simulink model "Coupled_Model_crosslinked_intext"  (R2016a)
settings: Solver=FixedStepDiscrete  StartTime=0  StopTime=1000  FixedStep=1  RelTol=1e-3
undefined symbols (not defined in the file or in its folder): DiscIntNeverNeededParam
libraries: simulink_extras x32
(part 1 of 3)
settings Model: Creator=bloomlab  LastModifiedBy=lawrimor
settings SolverCC: MaxOrder=2  AlgebraicLoopSolver=LineSearch
settings DataIOCC: LimitDataPoints=on  SaveFormat=Array  SignalLoggingSaveFormat=ModelDataLogs
settings OptimizationCC: ExpressionDepthLimit=2147483647  InitFltsAndDblsToZero=on
settings DebuggingCC: UnderspecifiedInitializationDetection=Classic  MergeDetectMultiDrivingBlocksExec=none  SolverPrmCheckMsg=warning  FcnCallInpInsideContextMsg=UseLocalSettings  UnconnectedOutputMsg=none  StateNameClashWarn=warning  StrictBusMsg=Warning
settings HardwareCC: ProdBitPerPointer=32  ProdLargestAtomicFloat=None  ProdIntDivRoundTo=Undefined  ProdEndianess=Unspecified  ProdWordSize=32  ProdHWDeviceType=32-bit Generic
settings ModelReferenceCC: ModelReferenceMinAlgLoopOccurrences=on  PropagateSignalLabelsOutOfModel=off
settings GRTTargetCC: CombineOutputUpdateFcns=off  GRTInterface=on
settings ConfigComp: CovModelRefEnable=Off

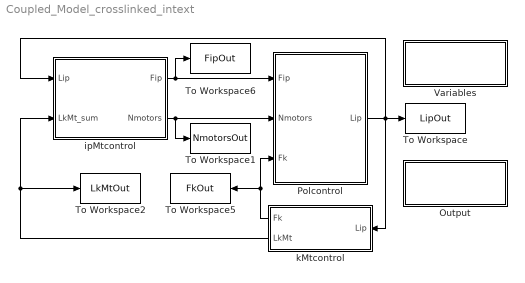
== system Coupled_Model_crosslinked_intext ==
  Output : Subsystem
  Polcontrol : Subsystem
  To Workspace : ToWorkspace  VariableName=LipOut  SampleTime=-1
  To Workspace1 : ToWorkspace  VariableName=NmotorsOut  SampleTime=-1
  To Workspace2 : ToWorkspace  VariableName=LkMtOut  SampleTime=-1
  To Workspace5 : ToWorkspace  VariableName=FkOut  SampleTime=-1
  To Workspace6 : ToWorkspace  VariableName=FipOut  SampleTime=-1
  Variables : Subsystem
  ipMtcontrol : Subsystem
  kMtcontrol : Subsystem
  wires:
  ipMtcontrol/2(Nmotors) -> Polcontrol/2(Nmotors), To Workspace1/1
  ipMtcontrol/1(Fip) -> Polcontrol/1(Fip), To Workspace6/1
  kMtcontrol/1(Fk) -> To Workspace5/1, Polcontrol/3(Fk)
  kMtcontrol/2(LkMt) -> ipMtcontrol/2(LkMt_sum), To Workspace2/1
  Polcontrol/1(Lip) -> kMtcontrol/1(Lip), ipMtcontrol/1(Lip), To Workspace/1

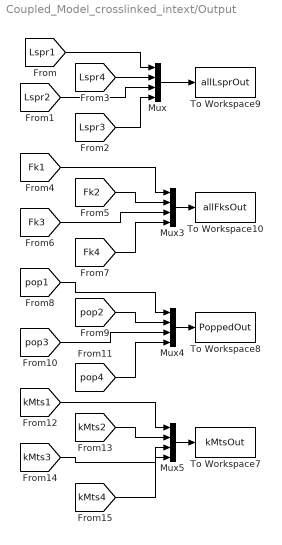
== system Coupled_Model_crosslinked_intext/Output ==
  Mux{,3..5} (4 alike) : Mux
  To Workspace10 : ToWorkspace  VariableName=allFksOut  SampleTime=-1
  To Workspace7 : ToWorkspace  VariableName=kMtsOut  SampleTime=-1
  To Workspace8 : ToWorkspace  VariableName=PoppedOut  SampleTime=-1
  To Workspace9 : ToWorkspace  VariableName=allLsprOut  SampleTime=-1
  wires:
  Mux/1 -> To Workspace9/1
  [Lspr1] -> Mux/1
  [Lspr4] -> Mux/2
  [Lspr2] -> Mux/3
  [Lspr3] -> Mux/4
  Mux3/1 -> To Workspace10/1
  [Fk1] -> Mux3/1
  [Fk2] -> Mux3/2
  [Fk3] -> Mux3/3
  [Fk4] -> Mux3/4
  Mux4/1 -> To Workspace8/1
  [pop1] -> Mux4/1
  [pop2] -> Mux4/2
  [pop3] -> Mux4/3
  [pop4] -> Mux4/4
  Mux5/1 -> To Workspace7/1
  [kMts1] -> Mux5/1
  [kMts2] -> Mux5/2
  [kMts3] -> Mux5/3
  [kMts4] -> Mux5/4

== system Coupled_Model_crosslinked_intext/Polcontrol ==
  Fip : Inport
  Nmotors : Inport  Port=2
  Fk : Inport  Port=3
  Discrete-Time Integrator : DiscreteIntegrator  InitialConditionSource=external  InitialCondition=1.5e-6  ICPrevOutput=DiscIntNeverNeededParam  ICPrevScaledInput=DiscIntNeverNeededParam
  Embedded MATLAB Function : MATLAB Function  TreatAsAtomicUnit=on
  Embedded MATLAB Function1 : MATLAB Function  TreatAsAtomicUnit=on
  Embedded MATLAB Function2 : MATLAB Function  TreatAsAtomicUnit=on
  Embedded MATLAB Function3 : MATLAB Function  TreatAsAtomicUnit=on
  Product : Product  RndMeth=Zero
  Sum : Sum
  Sum1 : Sum
  To Workspace4 : ToWorkspace  VariableName=vipOut  SampleTime=-1
  Lip : Outport
  wires:
  Embedded MATLAB Function/1(Vip) -> Product/1
  Fip/1 -> Sum/1
  Sum/1 -> Embedded MATLAB Function1/1(Fnet), Sum1/1
  Embedded MATLAB Function1/1(y) -> Embedded MATLAB Function/1(Fnet)
  Sum1/1 -> Embedded MATLAB Function3/1(Fnet)
  Embedded MATLAB Function3/1(y) -> Embedded MATLAB Function2/1(Fnet)
  Product/1 -> Sum1/2
  Embedded MATLAB Function2/1(Vip) -> Discrete-Time Integrator/1, To Workspace4/1
  Discrete-Time Integrator/1 -> Lip/1
  Nmotors/1 -> Embedded MATLAB Function1/2(Nmotors), Embedded MATLAB Function3/2(Nmotors)
  Fk/1 -> Sum/2
  [Cd] -> Product/2
  [Lip] -> Discrete-Time Integrator/2

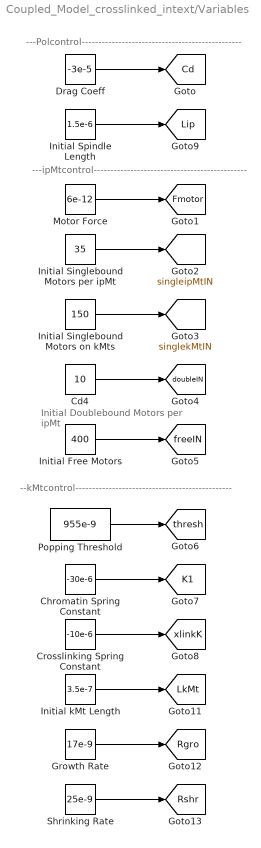
== system Coupled_Model_crosslinked_intext/Variables ==
  note: ---Polcontrol------------------------------------------------
  note: ---ipMtcontrol----------------------------------------------
  note: Initial Doublebound
      | Motors per ipMt
  note: --kMtcontrol-----------------------------------------------
  Cd4 : Constant  Value=10
  Chromatin Spring Constant : Constant  Value=-30e-6
  Crosslinking Spring Constant : Constant  Value=-10e-6
  Drag Coeff : Constant  Value=-3e-5
  Growth Rate : Constant  Value=17e-9
  Initial Free Motors : Constant  Value=400
  Initial Singlebound Motors on kMts : Constant  Value=150
  Initial Singlebound Motors per ipMt : Constant  Value=35
  Initial Spindle Length : Constant  Value=1.5e-6
  Initial kMt Length : Constant  Value=3.5e-7
  Motor Force : Constant  Value=6e-12
  Popping Threshold : Constant  Value=955e-9
  Shrinking Rate : Constant  Value=25e-9
  tag scope: Cd=global, Fmotor=global, K1=global, Lip=global, LkMt=global, Rgro=global, Rshr=global, doubleIN=global, freeIN=global, singleipMtIN=global, singlekMtIN=global, thresh=global, xlinkK=global
  wires:
  Drag Coeff/1 -> [Cd]
  Motor Force/1 -> [Fmotor]
  Initial Singlebound Motors per ipMt/1 -> [singleipMtIN]
  Initial Singlebound Motors on kMts/1 -> [singlekMtIN]
  Cd4/1 -> [doubleIN]
  Initial Free Motors/1 -> [freeIN]
  Popping Threshold/1 -> [thresh]
  Chromatin Spring Constant/1 -> [K1]
  Crosslinking Spring Constant/1 -> [xlinkK]
  Initial Spindle Length/1 -> [Lip]
  Initial kMt Length/1 -> [LkMt]
  Growth Rate/1 -> [Rgro]
  Shrinking Rate/1 -> [Rshr]

== system Coupled_Model_crosslinked_intext/ipMtcontrol ==
  note: Fk
  Lip : Inport
  LkMt_sum : Inport  Port=2
  Constant : Constant  Value=0.8e-6
  Embedded MATLAB Function1 : MATLAB Function
  Product : Product  RndMeth=Zero
  To Workspace3 : ToWorkspace  VariableName=LlapOut  SampleTime=-1
  Fip : Outport
  Nmotors : Outport  Port=2
  wires:
  Lip/1 -> Embedded MATLAB Function1/5(Lip)
  LkMt_sum/1 -> Embedded MATLAB Function1/7(LkMt)
  Product/1 -> Fip/1
  Embedded MATLAB Function1/1(Nmotors) -> Nmotors/1, Product/1
  [Fmotor] -> Product/2
  [singleipMtIN] -> Embedded MATLAB Function1/1(singleipMtIN)
  [singlekMtIN] -> Embedded MATLAB Function1/2(singlekMtIN)
  [doubleIN] -> Embedded MATLAB Function1/3(doubleIN)
  [freeIN] -> Embedded MATLAB Function1/4(freeIN)
  Constant/1 -> Embedded MATLAB Function1/6(Llap), To Workspace3/1

== system Coupled_Model_crosslinked_intext/kMtcontrol ==
  Lip : Inport
  Sum : Sum  Inputs=++++
  Sum1 : Sum  Inputs=++++
  kMtcontrol : Subsystem
  kMtcontrol1 : Subsystem
  kMtcontrol2 : Subsystem
  kMtcontrol3 : Subsystem
  Fk : Outport
  LkMt : Outport  Port=2
  wires:
  kMtcontrol/1(LkMt_sum) -> Sum/1
  kMtcontrol1/1(LkMt_sum) -> Sum/2
  kMtcontrol2/1(LkMt_sum) -> Sum/3
  kMtcontrol3/1(LkMt_sum) -> Sum/4
  kMtcontrol/2(Fk) -> Sum1/1
  kMtcontrol1/2(Fk) -> Sum1/2
  kMtcontrol2/2(Fk) -> Sum1/3
  kMtcontrol3/2(Fk) -> Sum1/4
  kMtcontrol/3(Lspring4) -> kMtcontrol1/2(Lspring4)
  kMtcontrol1/3(Lspring8) -> kMtcontrol2/2(Lspring8)
  kMtcontrol2/3(Lspring12) -> kMtcontrol3/2(Lspring12)
  kMtcontrol/4(Lspring1) -> kMtcontrol3/3(Lspring1)
  kMtcontrol3/4(Lspring13) -> kMtcontrol2/3(Lspring13)
  kMtcontrol2/4(Lspring9) -> kMtcontrol1/3(Lspring9)
  kMtcontrol1/4(Lspring5) -> kMtcontrol/3(Lspring5)
  kMtcontrol3/3(Lspring16) -> kMtcontrol/2(Lspring16)
  Lip/1 -> kMtcontrol2/1("Lip "), kMtcontrol3/1("Lip "), kMtcontrol/1("Lip "), kMtcontrol1/1("Lip ")
  Sum/1 -> LkMt/1
  Sum1/1 -> Fk/1

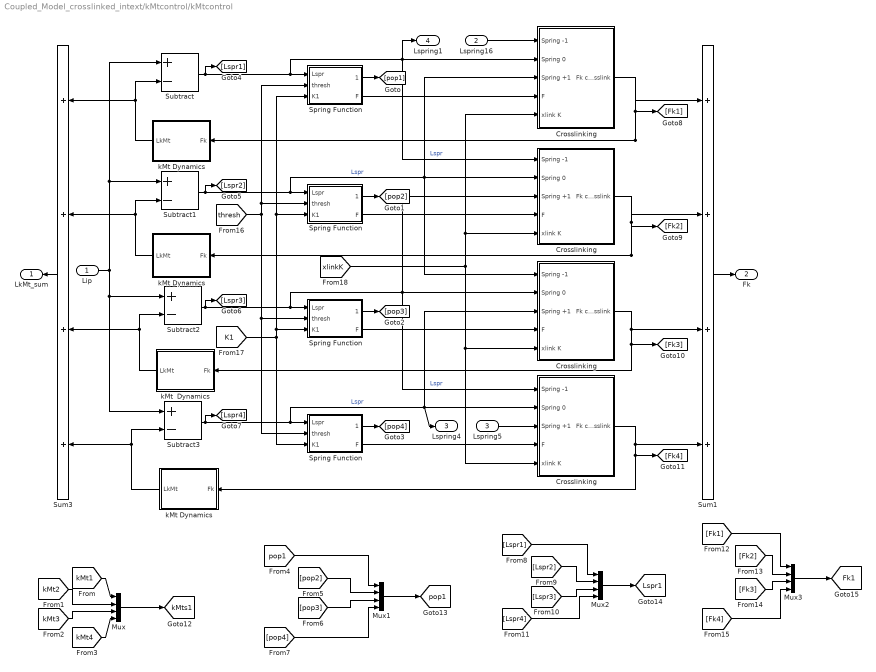
== system Coupled_Model_crosslinked_intext/kMtcontrol/kMtcontrol ==
  "Lip " : Inport
  Lspring16 : Inport  Port=2
  Lspring5 : Inport  Port=3
  " Crosslinking  " : Subsystem
  " Spring Function" : MATLAB Function  TreatAsAtomicUnit=on
  " Spring Function " : MATLAB Function  TreatAsAtomicUnit=on
  "Crosslinking " : Subsystem
  "Crosslinking  " : Subsystem
  "Crosslinking   " : Subsystem
  Mux{,1..3} (4 alike) : Mux
  Spring Function : MATLAB Function  TreatAsAtomicUnit=on
  "Spring Function " : MATLAB Function  TreatAsAtomicUnit=on
  Subtract{,1..3} (4 alike) : Sum  Inputs=+-
  Sum1 : Sum  Inputs=++++
  Sum3 : Sum  Inputs=++++
  kMt  Dynamics : Subsystem
  kMt Dynamics : Subsystem
  "kMt Dynamics " : Subsystem
  "kMt Dynamics  " : Subsystem
  LkMt_sum : Outport
  Fk : Outport  Port=2
  Lspring4 : Outport  Port=3
  Lspring1 : Outport  Port=4
  tag scope: Fk1=global, Lspr1=global, kMts1=global, pop1=global
  wires:
  "kMt Dynamics  "/1(LkMt) -> Subtract3/2, Sum3/4
  kMt  Dynamics/1(LkMt) -> Subtract2/2, Sum3/3
  "kMt Dynamics "/1(LkMt) -> Sum3/2, Subtract1/2
  kMt Dynamics/1(LkMt) -> Subtract/2, Sum3/1
  "Lip "/1 -> Subtract/1, Subtract1/1, Subtract2/1, Subtract3/1
  Sum1/1 -> Fk/1
  Subtract/1 -> [Lspr1], Spring Function/1(Lspr), "Crosslinking "/1(Spring -1), Lspring1/1, "Crosslinking  "/2(Spring 0)  "Lspr"
  Subtract1/1 -> [Lspr2], "Crosslinking  "/3(Spring +1), "Crosslinking "/2(Spring 0), " Crosslinking  "/1(Spring -1), "Spring Function "/1(Lspr)  "Lspr"
  Subtract2/1 -> [Lspr3], " Spring Function"/1(Lspr), " Crosslinking  "/2(Spring 0), "Crosslinking "/3(Spring +1), "Crosslinking   "/1(Spring -1)  "Lspr"
  Subtract3/1 -> [Lspr4], "Crosslinking   "/2(Spring 0), " Crosslinking  "/3(Spring +1), Lspring4/1, " Spring Function "/1(Lspr)  "Lspr"
  Spring Function/1(popped) -> [pop1]
  "Spring Function "/1(popped) -> [pop2]
  " Spring Function"/1(popped) -> [pop3]
  " Spring Function "/1(popped) -> [pop4]
  Mux/1 -> [kMts1]
  [kMt1] -> Mux/1
  [kMt2] -> Mux/2
  [kMt3] -> Mux/3
  [kMt4] -> Mux/4
  [pop1] -> Mux1/1
  [pop2] -> Mux1/2
  [pop3] -> Mux1/3
  [pop4] -> Mux1/4
  Mux1/1 -> [pop1]
  Mux2/1 -> [Lspr1]
  [Lspr1] -> Mux2/1
  [Lspr2] -> Mux2/2
  [Lspr3] -> Mux2/3
  [Lspr4] -> Mux2/4
  Mux3/1 -> [Fk1]
  [Fk1] -> Mux3/1
  [Fk2] -> Mux3/2
  [Fk3] -> Mux3/3
  [Fk4] -> Mux3/4
  Spring Function/2(F) -> "Crosslinking  "/4(F)
  "Crosslinking  "/1(Fk crosslink) -> kMt Dynamics/1(Fk), Sum1/1, [Fk1]
  "Spring Function "/2(F) -> "Crosslinking "/4(F)
  "Crosslinking "/1(Fk crosslink) -> Sum1/2, "kMt Dynamics "/1(Fk), [Fk2]
  " Spring Function"/2(F) -> " Crosslinking  "/4(F)
  " Crosslinking  "/1(Fk crosslink) -> [Fk3], kMt  Dynamics/1(Fk), Sum1/3
  " Spring Function "/2(F) -> "Crosslinking   "/4(F)
  "Crosslinking   "/1(Fk crosslink) -> Sum1/4, [Fk4], "kMt Dynamics  "/1(Fk)
  Lspring16/1 -> "Crosslinking  "/1(Spring -1)
  Lspring5/1 -> "Crosslinking   "/3(Spring +1)
  Sum3/1 -> LkMt_sum/1
  [thresh] -> "Spring Function "/2(thresh), Spring Function/2(thresh), " Spring Function"/2(thresh), " Spring Function "/2(thresh)
  [xlinkK] -> "Crosslinking "/5(xlink K), "Crosslinking  "/5(xlink K), " Crosslinking  "/5(xlink K), "Crosslinking   "/5(xlink K)
  [K1] -> " Spring Function "/3(K1), " Spring Function"/3(K1), "Spring Function "/3(K1), Spring Function/3(K1)

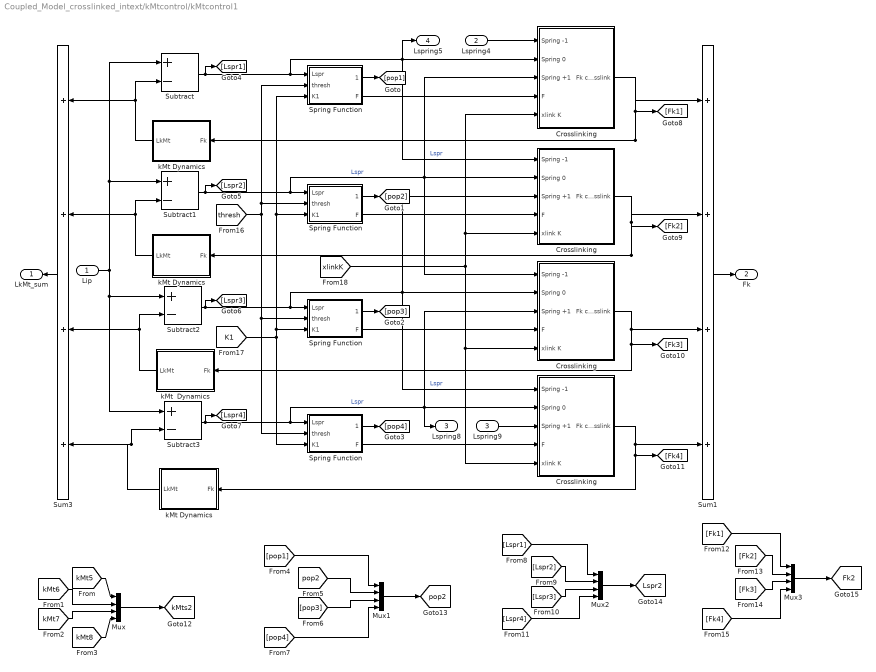
== system Coupled_Model_crosslinked_intext/kMtcontrol/kMtcontrol1 ==
  "Lip " : Inport
  Lspring4 : Inport  Port=2
  Lspring9 : Inport  Port=3
  " Crosslinking  " : Subsystem
  " Spring Function" : MATLAB Function  TreatAsAtomicUnit=on
  " Spring Function " : MATLAB Function  TreatAsAtomicUnit=on
  "Crosslinking " : Subsystem
  "Crosslinking  " : Subsystem
  "Crosslinking   " : Subsystem
  Mux{,1..3} (4 alike) : Mux
  Spring Function : MATLAB Function  TreatAsAtomicUnit=on
  "Spring Function " : MATLAB Function  TreatAsAtomicUnit=on
  Subtract{,1..3} (4 alike) : Sum  Inputs=+-
  Sum1 : Sum  Inputs=++++
  Sum3 : Sum  Inputs=++++
  kMt  Dynamics : Subsystem
  kMt Dynamics : Subsystem
  "kMt Dynamics " : Subsystem
  "kMt Dynamics  " : Subsystem
  LkMt_sum : Outport
  Fk : Outport  Port=2
  Lspring8 : Outport  Port=3
  Lspring5 : Outport  Port=4
  tag scope: Fk2=global, Lspr2=global, kMts2=global, pop2=global
  wires:
  [K1] -> " Spring Function "/3(K1), " Spring Function"/3(K1), "Spring Function "/3(K1), Spring Function/3(K1)
  [xlinkK] -> "Crosslinking "/5(xlink K), "Crosslinking  "/5(xlink K), " Crosslinking  "/5(xlink K), "Crosslinking   "/5(xlink K)
  [thresh] -> "Spring Function "/2(thresh), Spring Function/2(thresh), " Spring Function"/2(thresh), " Spring Function "/2(thresh)
  Sum3/1 -> LkMt_sum/1
  Lspring9/1 -> "Crosslinking   "/3(Spring +1)
  Lspring4/1 -> "Crosslinking  "/1(Spring -1)
  "Crosslinking   "/1(Fk crosslink) -> Sum1/4, [Fk4], "kMt Dynamics  "/1(Fk)
  " Spring Function "/2(F) -> "Crosslinking   "/4(F)
  " Crosslinking  "/1(Fk crosslink) -> [Fk3], kMt  Dynamics/1(Fk), Sum1/3
  " Spring Function"/2(F) -> " Crosslinking  "/4(F)
  "Crosslinking "/1(Fk crosslink) -> Sum1/2, "kMt Dynamics "/1(Fk), [Fk2]
  "Spring Function "/2(F) -> "Crosslinking "/4(F)
  "Crosslinking  "/1(Fk crosslink) -> Sum1/1, kMt Dynamics/1(Fk), [Fk1]
  Spring Function/2(F) -> "Crosslinking  "/4(F)
  [Fk4] -> Mux3/4
  [Fk3] -> Mux3/3
  [Fk2] -> Mux3/2
  [Fk1] -> Mux3/1
  Mux3/1 -> [Fk2]
  [Lspr4] -> Mux2/4
  [Lspr3] -> Mux2/3
  [Lspr2] -> Mux2/2
  [Lspr1] -> Mux2/1
  Mux2/1 -> [Lspr2]
  Mux1/1 -> [pop2]
  [pop4] -> Mux1/4
  [pop3] -> Mux1/3
  [pop2] -> Mux1/2
  [pop1] -> Mux1/1
  [kMt8] -> Mux/4
  [kMt7] -> Mux/3
  [kMt6] -> Mux/2
  [kMt5] -> Mux/1
  Mux/1 -> [kMts2]
  " Spring Function "/1(popped) -> [pop4]
  " Spring Function"/1(popped) -> [pop3]
  "Spring Function "/1(popped) -> [pop2]
  Spring Function/1(popped) -> [pop1]
  Subtract3/1 -> [Lspr4], "Crosslinking   "/2(Spring 0), " Crosslinking  "/3(Spring +1), Lspring8/1, " Spring Function "/1(Lspr)  "Lspr"
  Subtract2/1 -> [Lspr3], " Spring Function"/1(Lspr), " Crosslinking  "/2(Spring 0), "Crosslinking "/3(Spring +1), "Crosslinking   "/1(Spring -1)  "Lspr"
  Subtract1/1 -> [Lspr2], "Crosslinking  "/3(Spring +1), "Crosslinking "/2(Spring 0), " Crosslinking  "/1(Spring -1), "Spring Function "/1(Lspr)  "Lspr"
  Subtract/1 -> [Lspr1], Spring Function/1(Lspr), "Crosslinking "/1(Spring -1), Lspring5/1, "Crosslinking  "/2(Spring 0)  "Lspr"
  Sum1/1 -> Fk/1
  "Lip "/1 -> Subtract/1, Subtract1/1, Subtract2/1, Subtract3/1
  kMt Dynamics/1(LkMt) -> Subtract/2, Sum3/1
  "kMt Dynamics "/1(LkMt) -> Sum3/2, Subtract1/2
  kMt  Dynamics/1(LkMt) -> Subtract2/2, Sum3/3
  "kMt Dynamics  "/1(LkMt) -> Subtract3/2, Sum3/4

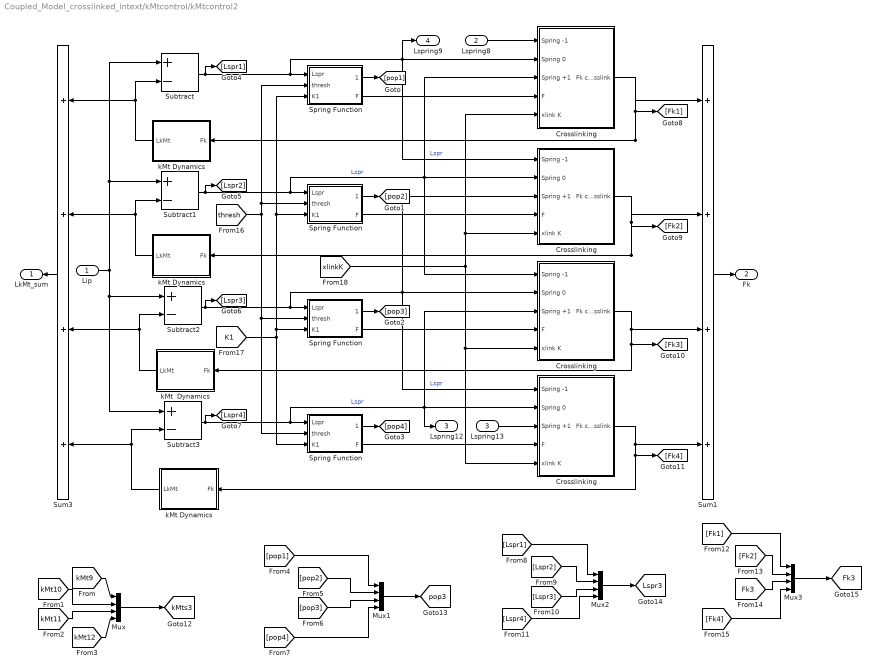
== system Coupled_Model_crosslinked_intext/kMtcontrol/kMtcontrol2 ==
  "Lip " : Inport
  Lspring8 : Inport  Port=2
  Lspring13 : Inport  Port=3
  " Crosslinking  " : Subsystem
  " Spring Function" : MATLAB Function  TreatAsAtomicUnit=on
  " Spring Function " : MATLAB Function  TreatAsAtomicUnit=on
  "Crosslinking " : Subsystem
  "Crosslinking  " : Subsystem
  "Crosslinking   " : Subsystem
  Mux{,1..3} (4 alike) : Mux
  Spring Function : MATLAB Function  TreatAsAtomicUnit=on
  "Spring Function " : MATLAB Function  TreatAsAtomicUnit=on
  Subtract{,1..3} (4 alike) : Sum  Inputs=+-
  Sum1 : Sum  Inputs=++++
  Sum3 : Sum  Inputs=++++
  kMt  Dynamics : Subsystem
  kMt Dynamics : Subsystem
  "kMt Dynamics " : Subsystem
  "kMt Dynamics  " : Subsystem
  LkMt_sum : Outport
  Fk : Outport  Port=2
  Lspring12 : Outport  Port=3
  Lspring9 : Outport  Port=4
  tag scope: Fk3=global, Lspr3=global, kMts3=global, pop3=global
  wires:
  "kMt Dynamics  "/1(LkMt) -> Subtract3/2, Sum3/4
  kMt  Dynamics/1(LkMt) -> Subtract2/2, Sum3/3
  "kMt Dynamics "/1(LkMt) -> Sum3/2, Subtract1/2
  kMt Dynamics/1(LkMt) -> Subtract/2, Sum3/1
  "Lip "/1 -> Subtract/1, Subtract1/1, Subtract2/1, Subtract3/1
  Sum1/1 -> Fk/1
  Subtract/1 -> [Lspr1], Spring Function/1(Lspr), "Crosslinking "/1(Spring -1), Lspring9/1, "Crosslinking  "/2(Spring 0)  "Lspr"
  Subtract1/1 -> [Lspr2], "Crosslinking  "/3(Spring +1), "Crosslinking "/2(Spring 0), " Crosslinking  "/1(Spring -1), "Spring Function "/1(Lspr)  "Lspr"
  Subtract2/1 -> [Lspr3], " Spring Function"/1(Lspr), " Crosslinking  "/2(Spring 0), "Crosslinking "/3(Spring +1), "Crosslinking   "/1(Spring -1)  "Lspr"
  Subtract3/1 -> [Lspr4], "Crosslinking   "/2(Spring 0), " Crosslinking  "/3(Spring +1), Lspring12/1, " Spring Function "/1(Lspr)  "Lspr"
  Spring Function/1(popped) -> [pop1]
  "Spring Function "/1(popped) -> [pop2]
  " Spring Function"/1(popped) -> [pop3]
  " Spring Function "/1(popped) -> [pop4]
  Mux/1 -> [kMts3]
  [kMt9] -> Mux/1
  [kMt10] -> Mux/2
  [kMt11] -> Mux/3
  [kMt12] -> Mux/4
  [pop1] -> Mux1/1
  [pop2] -> Mux1/2
  [pop3] -> Mux1/3
  [pop4] -> Mux1/4
  Mux1/1 -> [pop3]
  Mux2/1 -> [Lspr3]
  [Lspr1] -> Mux2/1
  [Lspr2] -> Mux2/2
  [Lspr3] -> Mux2/3
  [Lspr4] -> Mux2/4
  Mux3/1 -> [Fk3]
  [Fk1] -> Mux3/1
  [Fk2] -> Mux3/2
  [Fk3] -> Mux3/3
  [Fk4] -> Mux3/4
  Spring Function/2(F) -> "Crosslinking  "/4(F)
  "Crosslinking  "/1(Fk crosslink) -> Sum1/1, kMt Dynamics/1(Fk), [Fk1]
  "Spring Function "/2(F) -> "Crosslinking "/4(F)
  "Crosslinking "/1(Fk crosslink) -> Sum1/2, "kMt Dynamics "/1(Fk), [Fk2]
  " Spring Function"/2(F) -> " Crosslinking  "/4(F)
  " Crosslinking  "/1(Fk crosslink) -> [Fk3], kMt  Dynamics/1(Fk), Sum1/3
  " Spring Function "/2(F) -> "Crosslinking   "/4(F)
  "Crosslinking   "/1(Fk crosslink) -> Sum1/4, [Fk4], "kMt Dynamics  "/1(Fk)
  Lspring8/1 -> "Crosslinking  "/1(Spring -1)
  Lspring13/1 -> "Crosslinking   "/3(Spring +1)
  Sum3/1 -> LkMt_sum/1
  [thresh] -> "Spring Function "/2(thresh), Spring Function/2(thresh), " Spring Function"/2(thresh), " Spring Function "/2(thresh)
  [xlinkK] -> "Crosslinking "/5(xlink K), "Crosslinking  "/5(xlink K), " Crosslinking  "/5(xlink K), "Crosslinking   "/5(xlink K)
  [K1] -> " Spring Function "/3(K1), " Spring Function"/3(K1), "Spring Function "/3(K1), Spring Function/3(K1)

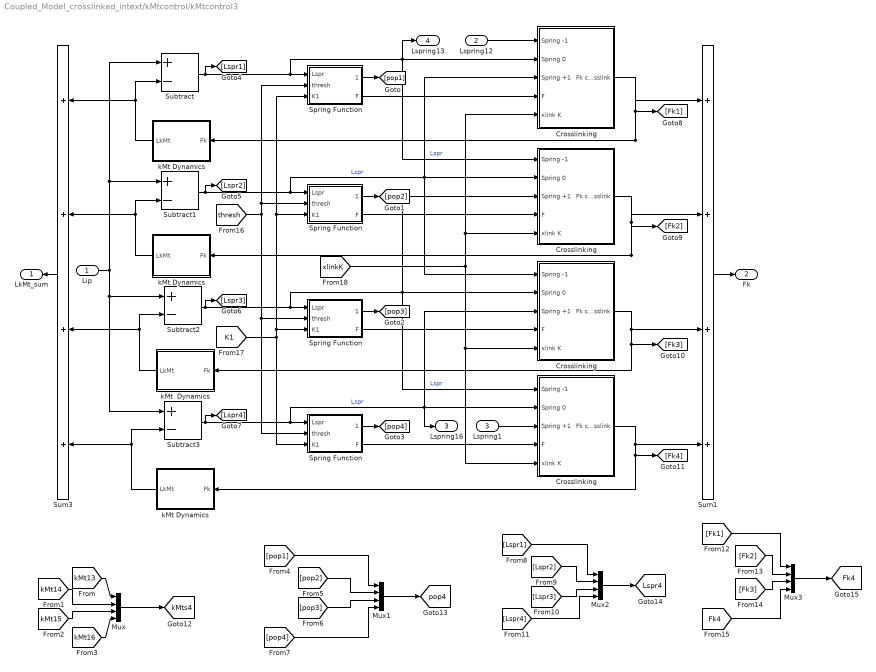
== system Coupled_Model_crosslinked_intext/kMtcontrol/kMtcontrol3 ==
  "Lip " : Inport
  Lspring12 : Inport  Port=2
  Lspring1 : Inport  Port=3
  " Crosslinking  " : Subsystem
  " Spring Function" : MATLAB Function  TreatAsAtomicUnit=on
  " Spring Function " : MATLAB Function  TreatAsAtomicUnit=on
  "Crosslinking " : Subsystem
  "Crosslinking  " : Subsystem
  "Crosslinking   " : Subsystem
  Mux{,1..3} (4 alike) : Mux
  Spring Function : MATLAB Function  TreatAsAtomicUnit=on
  "Spring Function " : MATLAB Function  TreatAsAtomicUnit=on
  Subtract{,1..3} (4 alike) : Sum  Inputs=+-
  Sum1 : Sum  Inputs=++++
  Sum3 : Sum  Inputs=++++
  kMt  Dynamics : Subsystem
  kMt Dynamics : Subsystem
  "kMt Dynamics " : Subsystem
  "kMt Dynamics  " : Subsystem
  LkMt_sum : Outport
  Fk : Outport  Port=2
  Lspring16 : Outport  Port=3
  Lspring13 : Outport  Port=4
  tag scope: Fk4=global, Lspr4=global, kMts4=global, pop4=global
  wires:
  "kMt Dynamics  "/1(LkMt) -> Subtract3/2, Sum3/4
  kMt  Dynamics/1(LkMt) -> Subtract2/2, Sum3/3
  "kMt Dynamics "/1(LkMt) -> Sum3/2, Subtract1/2
  kMt Dynamics/1(LkMt) -> Subtract/2, Sum3/1
  "Lip "/1 -> Subtract/1, Subtract1/1, Subtract2/1, Subtract3/1
  Sum1/1 -> Fk/1
  Subtract/1 -> [Lspr1], Spring Function/1(Lspr), "Crosslinking "/1(Spring -1), Lspring13/1, "Crosslinking  "/2(Spring 0)  "Lspr"
  Subtract1/1 -> [Lspr2], "Crosslinking  "/3(Spring +1), "Crosslinking "/2(Spring 0), " Crosslinking  "/1(Spring -1), "Spring Function "/1(Lspr)  "Lspr"
  Subtract2/1 -> [Lspr3], " Spring Function"/1(Lspr), " Crosslinking  "/2(Spring 0), "Crosslinking "/3(Spring +1), "Crosslinking   "/1(Spring -1)  "Lspr"
  Subtract3/1 -> [Lspr4], "Crosslinking   "/2(Spring 0), " Crosslinking  "/3(Spring +1), Lspring16/1, " Spring Function "/1(Lspr)  "Lspr"
  Spring Function/1(popped) -> [pop1]
  "Spring Function "/1(popped) -> [pop2]
  " Spring Function"/1(popped) -> [pop3]
  " Spring Function "/1(popped) -> [pop4]
  Mux/1 -> [kMts4]
  [kMt13] -> Mux/1
  [kMt14] -> Mux/2
  [kMt15] -> Mux/3
  [kMt16] -> Mux/4
  [pop1] -> Mux1/1
  [pop2] -> Mux1/2
  [pop3] -> Mux1/3
  [pop4] -> Mux1/4
  Mux1/1 -> [pop4]
  Mux2/1 -> [Lspr4]
  [Lspr1] -> Mux2/1
  [Lspr2] -> Mux2/2
  [Lspr3] -> Mux2/3
  [Lspr4] -> Mux2/4
  Mux3/1 -> [Fk4]
  [Fk1] -> Mux3/1
  [Fk2] -> Mux3/2
  [Fk3] -> Mux3/3
  [Fk4] -> Mux3/4
  Spring Function/2(F) -> "Crosslinking  "/4(F)
  "Crosslinking  "/1(Fk crosslink) -> Sum1/1, kMt Dynamics/1(Fk), [Fk1]
  "Spring Function "/2(F) -> "Crosslinking "/4(F)
  "Crosslinking "/1(Fk crosslink) -> Sum1/2, "kMt Dynamics "/1(Fk), [Fk2]
  " Spring Function"/2(F) -> " Crosslinking  "/4(F)
  " Crosslinking  "/1(Fk crosslink) -> [Fk3], kMt  Dynamics/1(Fk), Sum1/3
  " Spring Function "/2(F) -> "Crosslinking   "/4(F)
  "Crosslinking   "/1(Fk crosslink) -> Sum1/4, [Fk4], "kMt Dynamics  "/1(Fk)
  Lspring12/1 -> "Crosslinking  "/1(Spring -1)
  Lspring1/1 -> "Crosslinking   "/3(Spring +1)
  Sum3/1 -> LkMt_sum/1
  [thresh] -> "Spring Function "/2(thresh), Spring Function/2(thresh), " Spring Function"/2(thresh), " Spring Function "/2(thresh)
  [xlinkK] -> "Crosslinking "/5(xlink K), "Crosslinking  "/5(xlink K), " Crosslinking  "/5(xlink K), "Crosslinking   "/5(xlink K)
  [K1] -> " Spring Function "/3(K1), " Spring Function"/3(K1), "Spring Function "/3(K1), Spring Function/3(K1)

== system Coupled_Model_crosslinked_intext/kMtcontrol/kMtcontrol/ Crosslinking   ==
  Spring -1 : Inport
  Spring 0 : Inport  Port=2
  Spring +1 : Inport  Port=3
  F : Inport  Port=4
  xlink K : Inport  Port=5
  Product : Product  RndMeth=Zero
  Product1 : Product  RndMeth=Zero
  Subtract1 : Sum  Inputs=+-
  Subtract3 : Sum  Inputs=-++
  Subtract4 : Sum  Inputs=+-
  Fk crosslink : Outport
  wires:
  Spring -1/1 -> Subtract1/1
  Spring 0/1 -> Subtract1/2, Subtract4/1
  Spring +1/1 -> Subtract4/2
  xlink K/1 -> Product/2, Product1/1
  Subtract1/1 -> Product/1
  Subtract4/1 -> Product1/2
  Product/1 -> Subtract3/1
  F/1 -> Subtract3/2
  Product1/1 -> Subtract3/3
  Subtract3/1 -> Fk crosslink/1

== system Coupled_Model_crosslinked_intext/kMtcontrol/kMtcontrol/Crosslinking  ==
  Spring -1 : Inport
  Spring 0 : Inport  Port=2
  Spring +1 : Inport  Port=3
  F : Inport  Port=4
  xlink K : Inport  Port=5
  Product : Product  RndMeth=Zero
  Product1 : Product  RndMeth=Zero
  Subtract1 : Sum  Inputs=+-
  Subtract3 : Sum  Inputs=-++
  Subtract4 : Sum  Inputs=+-
  Fk crosslink : Outport
  wires:
  Spring -1/1 -> Subtract1/1
  Spring 0/1 -> Subtract1/2, Subtract4/1
  Spring +1/1 -> Subtract4/2
  xlink K/1 -> Product/2, Product1/1
  Subtract1/1 -> Product/1
  Subtract4/1 -> Product1/2
  Product/1 -> Subtract3/1
  F/1 -> Subtract3/2
  Product1/1 -> Subtract3/3
  Subtract3/1 -> Fk crosslink/1

== system Coupled_Model_crosslinked_intext/kMtcontrol/kMtcontrol/Crosslinking   ==
  Spring -1 : Inport
  Spring 0 : Inport  Port=2
  Spring +1 : Inport  Port=3
  F : Inport  Port=4
  xlink K : Inport  Port=5
  Product : Product  RndMeth=Zero
  Product1 : Product  RndMeth=Zero
  Subtract1 : Sum  Inputs=+-
  Subtract3 : Sum  Inputs=-++
  Subtract4 : Sum  Inputs=+-
  Fk crosslink : Outport
  wires:
  Spring -1/1 -> Subtract1/1
  Spring 0/1 -> Subtract1/2, Subtract4/1
  Spring +1/1 -> Subtract4/2
  xlink K/1 -> Product/2, Product1/1
  Subtract1/1 -> Product/1
  Subtract4/1 -> Product1/2
  Product/1 -> Subtract3/1
  F/1 -> Subtract3/2
  Product1/1 -> Subtract3/3
  Subtract3/1 -> Fk crosslink/1

== system Coupled_Model_crosslinked_intext/kMtcontrol/kMtcontrol/Crosslinking    ==
  Spring -1 : Inport
  Spring 0 : Inport  Port=2
  Spring +1 : Inport  Port=3
  F : Inport  Port=4
  xlink K : Inport  Port=5
  Product : Product  RndMeth=Zero
  Product1 : Product  RndMeth=Zero
  Subtract1 : Sum  Inputs=+-
  Subtract3 : Sum  Inputs=-++
  Subtract4 : Sum  Inputs=+-
  Fk crosslink : Outport
  wires:
  Spring -1/1 -> Subtract1/1
  Spring 0/1 -> Subtract1/2, Subtract4/1
  Spring +1/1 -> Subtract4/2
  xlink K/1 -> Product/2, Product1/1
  Subtract1/1 -> Product/1
  Subtract4/1 -> Product1/2
  Product/1 -> Subtract3/1
  F/1 -> Subtract3/2
  Product1/1 -> Subtract3/3
  Subtract3/1 -> Fk crosslink/1

== system Coupled_Model_crosslinked_intext/kMtcontrol/kMtcontrol/kMt  Dynamics ==
  Fk : Inport
  Add : Sum  Inputs=-+
  Add1 : Sum  Inputs=-+
  Add2 : Sum
  Discrete-Time Integrator : DiscreteIntegrator  InitialConditionSource=external  ICPrevOutput=DiscIntNeverNeededParam  ICPrevScaledInput=DiscIntNeverNeededParam
  Discrete-Time Integrator1 : DiscreteIntegrator  InitialConditionSource=external  ICPrevOutput=DiscIntNeverNeededParam  ICPrevScaledInput=DiscIntNeverNeededParam
  Mux : Mux  Inputs=2
  Product{1..4} (4 alike) : Product  RndMeth=Zero
  kMtState : Subsystem
  LkMt : Outport
  tag scope: kMt3=global
  wires:
  Fk/1 -> kMtState/2(Fspr)
  kMtState/2(RLeft) -> Product2/1
  Product1/1 -> Add/1
  Product2/1 -> Add/2
  Product3/1 -> Add1/2
  Product4/1 -> Add1/1
  kMtState/4(RRight) -> Product3/1
  kMtState/1(CLeft) -> Product1/1
  Add/1 -> Discrete-Time Integrator/1  "glkMt"
  Add1/1 -> Discrete-Time Integrator1/1  "grkMt"
  Discrete-Time Integrator1/1 -> Add2/2, kMtState/3(LrkMt), Mux/2
  Discrete-Time Integrator/1 -> Add2/1, kMtState/1(LlkMt), Mux/1
  Add2/1 -> LkMt/1
  kMtState/3(CRight) -> Product4/1
  [Rgro] -> Product2/2, Product3/2
  [Rshr] -> Product1/2, Product4/2
  Mux/1 -> [kMt3]
  [LkMt] -> Discrete-Time Integrator/2
  [LkMt] -> Discrete-Time Integrator1/2

== system Coupled_Model_crosslinked_intext/kMtcontrol/kMtcontrol/kMt Dynamics ==
  Fk : Inport
  Add : Sum  Inputs=-+
  Add1 : Sum  Inputs=-+
  Add2 : Sum
  Discrete-Time Integrator : DiscreteIntegrator  InitialConditionSource=external  ICPrevOutput=DiscIntNeverNeededParam  ICPrevScaledInput=DiscIntNeverNeededParam
  Discrete-Time Integrator1 : DiscreteIntegrator  InitialConditionSource=external  ICPrevOutput=DiscIntNeverNeededParam  ICPrevScaledInput=DiscIntNeverNeededParam
  Mux : Mux  Inputs=2
  Product{1..4} (4 alike) : Product  RndMeth=Zero
  kMtState : Subsystem
  LkMt : Outport
  tag scope: kMt1=global
  wires:
  Fk/1 -> kMtState/2(Fspr)
  kMtState/2(RLeft) -> Product2/1
  Product1/1 -> Add/1
  Product2/1 -> Add/2
  Product3/1 -> Add1/2
  Product4/1 -> Add1/1
  kMtState/4(RRight) -> Product3/1
  kMtState/1(CLeft) -> Product1/1
  Add/1 -> Discrete-Time Integrator/1  "glkMt"
  Add1/1 -> Discrete-Time Integrator1/1  "grkMt"
  Discrete-Time Integrator1/1 -> Add2/2, kMtState/3(LrkMt), Mux/2
  Discrete-Time Integrator/1 -> Add2/1, kMtState/1(LlkMt), Mux/1
  Add2/1 -> LkMt/1
  kMtState/3(CRight) -> Product4/1
  [Rgro] -> Product2/2, Product3/2
  [Rshr] -> Product1/2, Product4/2
  Mux/1 -> [kMt1]
  [LkMt] -> Discrete-Time Integrator/2
  [LkMt] -> Discrete-Time Integrator1/2

== system Coupled_Model_crosslinked_intext/kMtcontrol/kMtcontrol/kMt Dynamics  ==
  Fk : Inport
  Add : Sum  Inputs=-+
  Add1 : Sum  Inputs=-+
  Add2 : Sum
  Discrete-Time Integrator : DiscreteIntegrator  InitialConditionSource=external  ICPrevOutput=DiscIntNeverNeededParam  ICPrevScaledInput=DiscIntNeverNeededParam
  Discrete-Time Integrator1 : DiscreteIntegrator  InitialConditionSource=external  ICPrevOutput=DiscIntNeverNeededParam  ICPrevScaledInput=DiscIntNeverNeededParam
  Mux : Mux  Inputs=2
  Product{1..4} (4 alike) : Product  RndMeth=Zero
  kMtState : Subsystem
  LkMt : Outport
  tag scope: kMt2=global
  wires:
  Fk/1 -> kMtState/2(Fspr)
  kMtState/2(RLeft) -> Product2/1
  Product1/1 -> Add/1
  Product2/1 -> Add/2
  Product3/1 -> Add1/2
  Product4/1 -> Add1/1
  kMtState/4(RRight) -> Product3/1
  kMtState/1(CLeft) -> Product1/1
  Add/1 -> Discrete-Time Integrator/1  "glkMt"
  Add1/1 -> Discrete-Time Integrator1/1  "grkMt"
  Discrete-Time Integrator1/1 -> Add2/2, kMtState/3(LrkMt), Mux/2
  Discrete-Time Integrator/1 -> Add2/1, kMtState/1(LlkMt), Mux/1
  Add2/1 -> LkMt/1
  kMtState/3(CRight) -> Product4/1
  [Rgro] -> Product2/2, Product3/2
  [Rshr] -> Product1/2, Product4/2
  Mux/1 -> [kMt2]
  [LkMt] -> Discrete-Time Integrator/2
  [LkMt] -> Discrete-Time Integrator1/2

== system Coupled_Model_crosslinked_intext/kMtcontrol/kMtcontrol/kMt Dynamics   ==
  Fk : Inport
  Add : Sum  Inputs=-+
  Add1 : Sum  Inputs=-+
  Add2 : Sum
  Discrete-Time Integrator : DiscreteIntegrator  InitialConditionSource=external  ICPrevOutput=DiscIntNeverNeededParam  ICPrevScaledInput=DiscIntNeverNeededParam
  Discrete-Time Integrator1 : DiscreteIntegrator  InitialConditionSource=external  ICPrevOutput=DiscIntNeverNeededParam  ICPrevScaledInput=DiscIntNeverNeededParam
  Mux : Mux  Inputs=2
  Product{1..4} (4 alike) : Product  RndMeth=Zero
  kMtState : Subsystem
  LkMt : Outport
  tag scope: kMt4=global
  wires:
  Fk/1 -> kMtState/2(Fspr)
  kMtState/2(RLeft) -> Product2/1
  Product1/1 -> Add/1
  Product2/1 -> Add/2
  Product3/1 -> Add1/2
  Product4/1 -> Add1/1
  kMtState/4(RRight) -> Product3/1
  kMtState/1(CLeft) -> Product1/1
  Add/1 -> Discrete-Time Integrator/1  "glkMt"
  Add1/1 -> Discrete-Time Integrator1/1  "grkMt"
  Discrete-Time Integrator1/1 -> Add2/2, kMtState/3(LrkMt), Mux/2
  Discrete-Time Integrator/1 -> Add2/1, kMtState/1(LlkMt), Mux/1
  Add2/1 -> LkMt/1
  kMtState/3(CRight) -> Product4/1
  [Rgro] -> Product2/2, Product3/2
  [Rshr] -> Product1/2, Product4/2
  Mux/1 -> [kMt4]
  [LkMt] -> Discrete-Time Integrator/2
  [LkMt] -> Discrete-Time Integrator1/2

== system Coupled_Model_crosslinked_intext/kMtcontrol/kMtcontrol1/ Crosslinking   ==
  Spring -1 : Inport
  Spring 0 : Inport  Port=2
  Spring +1 : Inport  Port=3
  F : Inport  Port=4
  xlink K : Inport  Port=5
  Product : Product  RndMeth=Zero
  Product1 : Product  RndMeth=Zero
  Subtract1 : Sum  Inputs=+-
  Subtract3 : Sum  Inputs=-++
  Subtract4 : Sum  Inputs=+-
  Fk crosslink : Outport
  wires:
  Spring -1/1 -> Subtract1/1
  Spring 0/1 -> Subtract1/2, Subtract4/1
  Spring +1/1 -> Subtract4/2
  xlink K/1 -> Product/2, Product1/1
  Subtract1/1 -> Product/1
  Subtract4/1 -> Product1/2
  Product/1 -> Subtract3/1
  F/1 -> Subtract3/2
  Product1/1 -> Subtract3/3
  Subtract3/1 -> Fk crosslink/1

== system Coupled_Model_crosslinked_intext/kMtcontrol/kMtcontrol1/Crosslinking  ==
  Spring -1 : Inport
  Spring 0 : Inport  Port=2
  Spring +1 : Inport  Port=3
  F : Inport  Port=4
  xlink K : Inport  Port=5
  Product : Product  RndMeth=Zero
  Product1 : Product  RndMeth=Zero
  Subtract1 : Sum  Inputs=+-
  Subtract3 : Sum  Inputs=-++
  Subtract4 : Sum  Inputs=+-
  Fk crosslink : Outport
  wires:
  Spring -1/1 -> Subtract1/1
  Spring 0/1 -> Subtract1/2, Subtract4/1
  Spring +1/1 -> Subtract4/2
  xlink K/1 -> Product/2, Product1/1
  Subtract1/1 -> Product/1
  Subtract4/1 -> Product1/2
  Product/1 -> Subtract3/1
  F/1 -> Subtract3/2
  Product1/1 -> Subtract3/3
  Subtract3/1 -> Fk crosslink/1

== system Coupled_Model_crosslinked_intext/kMtcontrol/kMtcontrol1/Crosslinking   ==
  Spring -1 : Inport
  Spring 0 : Inport  Port=2
  Spring +1 : Inport  Port=3
  F : Inport  Port=4
  xlink K : Inport  Port=5
  Product : Product  RndMeth=Zero
  Product1 : Product  RndMeth=Zero
  Subtract1 : Sum  Inputs=+-
  Subtract3 : Sum  Inputs=-++
  Subtract4 : Sum  Inputs=+-
  Fk crosslink : Outport
  wires:
  Spring -1/1 -> Subtract1/1
  Spring 0/1 -> Subtract1/2, Subtract4/1
  Spring +1/1 -> Subtract4/2
  xlink K/1 -> Product/2, Product1/1
  Subtract1/1 -> Product/1
  Subtract4/1 -> Product1/2
  Product/1 -> Subtract3/1
  F/1 -> Subtract3/2
  Product1/1 -> Subtract3/3
  Subtract3/1 -> Fk crosslink/1

== system Coupled_Model_crosslinked_intext/kMtcontrol/kMtcontrol1/Crosslinking    ==
  Spring -1 : Inport
  Spring 0 : Inport  Port=2
  Spring +1 : Inport  Port=3
  F : Inport  Port=4
  xlink K : Inport  Port=5
  Product : Product  RndMeth=Zero
  Product1 : Product  RndMeth=Zero
  Subtract1 : Sum  Inputs=+-
  Subtract3 : Sum  Inputs=-++
  Subtract4 : Sum  Inputs=+-
  Fk crosslink : Outport
  wires:
  Spring -1/1 -> Subtract1/1
  Spring 0/1 -> Subtract1/2, Subtract4/1
  Spring +1/1 -> Subtract4/2
  xlink K/1 -> Product/2, Product1/1
  Subtract1/1 -> Product/1
  Subtract4/1 -> Product1/2
  Product/1 -> Subtract3/1
  F/1 -> Subtract3/2
  Product1/1 -> Subtract3/3
  Subtract3/1 -> Fk crosslink/1

== system Coupled_Model_crosslinked_intext/kMtcontrol/kMtcontrol1/kMt  Dynamics ==
  Fk : Inport
  Add : Sum  Inputs=-+
  Add1 : Sum  Inputs=-+
  Add2 : Sum
  Discrete-Time Integrator : DiscreteIntegrator  InitialConditionSource=external  ICPrevOutput=DiscIntNeverNeededParam  ICPrevScaledInput=DiscIntNeverNeededParam
  Discrete-Time Integrator1 : DiscreteIntegrator  InitialConditionSource=external  ICPrevOutput=DiscIntNeverNeededParam  ICPrevScaledInput=DiscIntNeverNeededParam
  Mux : Mux  Inputs=2
  Product{1..4} (4 alike) : Product  RndMeth=Zero
  kMtState : Subsystem
  LkMt : Outport
  tag scope: kMt7=global
  wires:
  Fk/1 -> kMtState/2(Fspr)
  kMtState/2(RLeft) -> Product2/1
  Product1/1 -> Add/1
  Product2/1 -> Add/2
  Product3/1 -> Add1/2
  Product4/1 -> Add1/1
  kMtState/4(RRight) -> Product3/1
  kMtState/1(CLeft) -> Product1/1
  Add/1 -> Discrete-Time Integrator/1  "glkMt"
  Add1/1 -> Discrete-Time Integrator1/1  "grkMt"
  Discrete-Time Integrator1/1 -> Add2/2, kMtState/3(LrkMt), Mux/2
  Discrete-Time Integrator/1 -> Add2/1, kMtState/1(LlkMt), Mux/1
  Add2/1 -> LkMt/1
  kMtState/3(CRight) -> Product4/1
  [Rgro] -> Product2/2, Product3/2
  [Rshr] -> Product1/2, Product4/2
  Mux/1 -> [kMt7]
  [LkMt] -> Discrete-Time Integrator/2
  [LkMt] -> Discrete-Time Integrator1/2

== system Coupled_Model_crosslinked_intext/kMtcontrol/kMtcontrol1/kMt Dynamics ==
  Fk : Inport
  Add : Sum  Inputs=-+
  Add1 : Sum  Inputs=-+
  Add2 : Sum
  Discrete-Time Integrator : DiscreteIntegrator  InitialConditionSource=external  ICPrevOutput=DiscIntNeverNeededParam  ICPrevScaledInput=DiscIntNeverNeededParam
  Discrete-Time Integrator1 : DiscreteIntegrator  InitialConditionSource=external  ICPrevOutput=DiscIntNeverNeededParam  ICPrevScaledInput=DiscIntNeverNeededParam
  Mux : Mux  Inputs=2
  Product{1..4} (4 alike) : Product  RndMeth=Zero
  kMtState : Subsystem
  LkMt : Outport
  tag scope: kMt5=global
  wires:
  Fk/1 -> kMtState/2(Fspr)
  kMtState/2(RLeft) -> Product2/1
  Product1/1 -> Add/1
  Product2/1 -> Add/2
  Product3/1 -> Add1/2
  Product4/1 -> Add1/1
  kMtState/4(RRight) -> Product3/1
  kMtState/1(CLeft) -> Product1/1
  Add/1 -> Discrete-Time Integrator/1  "glkMt"
  Add1/1 -> Discrete-Time Integrator1/1  "grkMt"
  Discrete-Time Integrator1/1 -> Add2/2, kMtState/3(LrkMt), Mux/2
  Discrete-Time Integrator/1 -> Add2/1, kMtState/1(LlkMt), Mux/1
  Add2/1 -> LkMt/1
  kMtState/3(CRight) -> Product4/1
  [Rgro] -> Product2/2, Product3/2
  [Rshr] -> Product1/2, Product4/2
  Mux/1 -> [kMt5]
  [LkMt] -> Discrete-Time Integrator/2
  [LkMt] -> Discrete-Time Integrator1/2

== system Coupled_Model_crosslinked_intext/kMtcontrol/kMtcontrol1/kMt Dynamics  ==
  Fk : Inport
  Add : Sum  Inputs=-+
  Add1 : Sum  Inputs=-+
  Add2 : Sum
  Discrete-Time Integrator : DiscreteIntegrator  InitialConditionSource=external  ICPrevOutput=DiscIntNeverNeededParam  ICPrevScaledInput=DiscIntNeverNeededParam
  Discrete-Time Integrator1 : DiscreteIntegrator  InitialConditionSource=external  ICPrevOutput=DiscIntNeverNeededParam  ICPrevScaledInput=DiscIntNeverNeededParam
  Mux : Mux  Inputs=2
  Product{1..4} (4 alike) : Product  RndMeth=Zero
  kMtState : Subsystem
  LkMt : Outport
  tag scope: kMt6=global
  wires:
  Fk/1 -> kMtState/2(Fspr)
  kMtState/2(RLeft) -> Product2/1
  Product1/1 -> Add/1
  Product2/1 -> Add/2
  Product3/1 -> Add1/2
  Product4/1 -> Add1/1
  kMtState/4(RRight) -> Product3/1
  kMtState/1(CLeft) -> Product1/1
  Add/1 -> Discrete-Time Integrator/1  "glkMt"
  Add1/1 -> Discrete-Time Integrator1/1  "grkMt"
  Discrete-Time Integrator1/1 -> Add2/2, kMtState/3(LrkMt), Mux/2
  Discrete-Time Integrator/1 -> Add2/1, kMtState/1(LlkMt), Mux/1
  Add2/1 -> LkMt/1
  kMtState/3(CRight) -> Product4/1
  [Rgro] -> Product2/2, Product3/2
  [Rshr] -> Product1/2, Product4/2
  Mux/1 -> [kMt6]
  [LkMt] -> Discrete-Time Integrator/2
  [LkMt] -> Discrete-Time Integrator1/2

== system Coupled_Model_crosslinked_intext/kMtcontrol/kMtcontrol1/kMt Dynamics   ==
  Fk : Inport
  Add : Sum  Inputs=-+
  Add1 : Sum  Inputs=-+
  Add2 : Sum
  Discrete-Time Integrator : DiscreteIntegrator  InitialConditionSource=external  ICPrevOutput=DiscIntNeverNeededParam  ICPrevScaledInput=DiscIntNeverNeededParam
  Discrete-Time Integrator1 : DiscreteIntegrator  InitialConditionSource=external  ICPrevOutput=DiscIntNeverNeededParam  ICPrevScaledInput=DiscIntNeverNeededParam
  Mux : Mux  Inputs=2
  Product{1..4} (4 alike) : Product  RndMeth=Zero
  kMtState : Subsystem
  LkMt : Outport
  tag scope: kMt8=global
  wires:
  Fk/1 -> kMtState/2(Fspr)
  kMtState/2(RLeft) -> Product2/1
  Product1/1 -> Add/1
  Product2/1 -> Add/2
  Product3/1 -> Add1/2
  Product4/1 -> Add1/1
  kMtState/4(RRight) -> Product3/1
  kMtState/1(CLeft) -> Product1/1
  Add/1 -> Discrete-Time Integrator/1  "glkMt"
  Add1/1 -> Discrete-Time Integrator1/1  "grkMt"
  Discrete-Time Integrator1/1 -> Add2/2, kMtState/3(LrkMt), Mux/2
  Discrete-Time Integrator/1 -> Add2/1, kMtState/1(LlkMt), Mux/1
  Add2/1 -> LkMt/1
  kMtState/3(CRight) -> Product4/1
  [Rgro] -> Product2/2, Product3/2
  [Rshr] -> Product1/2, Product4/2
  Mux/1 -> [kMt8]
  [LkMt] -> Discrete-Time Integrator/2
  [LkMt] -> Discrete-Time Integrator1/2

== system Coupled_Model_crosslinked_intext/kMtcontrol/kMtcontrol2/ Crosslinking   ==
  Spring -1 : Inport
  Spring 0 : Inport  Port=2
  Spring +1 : Inport  Port=3
  F : Inport  Port=4
  xlink K : Inport  Port=5
  Product : Product  RndMeth=Zero
  Product1 : Product  RndMeth=Zero
  Subtract1 : Sum  Inputs=+-
  Subtract3 : Sum  Inputs=-++
  Subtract4 : Sum  Inputs=+-
  Fk crosslink : Outport
  wires:
  Spring -1/1 -> Subtract1/1
  Spring 0/1 -> Subtract1/2, Subtract4/1
  Spring +1/1 -> Subtract4/2
  xlink K/1 -> Product/2, Product1/1
  Subtract1/1 -> Product/1
  Subtract4/1 -> Product1/2
  Product/1 -> Subtract3/1
  F/1 -> Subtract3/2
  Product1/1 -> Subtract3/3
  Subtract3/1 -> Fk crosslink/1

== system Coupled_Model_crosslinked_intext/kMtcontrol/kMtcontrol2/Crosslinking  ==
  Spring -1 : Inport
  Spring 0 : Inport  Port=2
  Spring +1 : Inport  Port=3
  F : Inport  Port=4
  xlink K : Inport  Port=5
  Product : Product  RndMeth=Zero
  Product1 : Product  RndMeth=Zero
  Subtract1 : Sum  Inputs=+-
  Subtract3 : Sum  Inputs=-++
  Subtract4 : Sum  Inputs=+-
  Fk crosslink : Outport
  wires:
  Spring -1/1 -> Subtract1/1
  Spring 0/1 -> Subtract1/2, Subtract4/1
  Spring +1/1 -> Subtract4/2
  xlink K/1 -> Product/2, Product1/1
  Subtract1/1 -> Product/1
  Subtract4/1 -> Product1/2
  Product/1 -> Subtract3/1
  F/1 -> Subtract3/2
  Product1/1 -> Subtract3/3
  Subtract3/1 -> Fk crosslink/1

== system Coupled_Model_crosslinked_intext/kMtcontrol/kMtcontrol2/Crosslinking   ==
  Spring -1 : Inport
  Spring 0 : Inport  Port=2
  Spring +1 : Inport  Port=3
  F : Inport  Port=4
  xlink K : Inport  Port=5
  Product : Product  RndMeth=Zero
  Product1 : Product  RndMeth=Zero
  Subtract1 : Sum  Inputs=+-
  Subtract3 : Sum  Inputs=-++
  Subtract4 : Sum  Inputs=+-
  Fk crosslink : Outport
  wires:
  Spring -1/1 -> Subtract1/1
  Spring 0/1 -> Subtract1/2, Subtract4/1
  Spring +1/1 -> Subtract4/2
  xlink K/1 -> Product/2, Product1/1
  Subtract1/1 -> Product/1
  Subtract4/1 -> Product1/2
  Product/1 -> Subtract3/1
  F/1 -> Subtract3/2
  Product1/1 -> Subtract3/3
  Subtract3/1 -> Fk crosslink/1

== system Coupled_Model_crosslinked_intext/kMtcontrol/kMtcontrol2/Crosslinking    ==
  Spring -1 : Inport
  Spring 0 : Inport  Port=2
  Spring +1 : Inport  Port=3
  F : Inport  Port=4
  xlink K : Inport  Port=5
  Product : Product  RndMeth=Zero
  Product1 : Product  RndMeth=Zero
  Subtract1 : Sum  Inputs=+-
  Subtract3 : Sum  Inputs=-++
  Subtract4 : Sum  Inputs=+-
  Fk crosslink : Outport
  wires:
  Spring -1/1 -> Subtract1/1
  Spring 0/1 -> Subtract1/2, Subtract4/1
  Spring +1/1 -> Subtract4/2
  xlink K/1 -> Product/2, Product1/1
  Subtract1/1 -> Product/1
  Subtract4/1 -> Product1/2
  Product/1 -> Subtract3/1
  F/1 -> Subtract3/2
  Product1/1 -> Subtract3/3
  Subtract3/1 -> Fk crosslink/1

== system Coupled_Model_crosslinked_intext/kMtcontrol/kMtcontrol2/kMt  Dynamics ==
  Fk : Inport
  Add : Sum  Inputs=-+
  Add1 : Sum  Inputs=-+
  Add2 : Sum
  Discrete-Time Integrator : DiscreteIntegrator  InitialConditionSource=external  ICPrevOutput=DiscIntNeverNeededParam  ICPrevScaledInput=DiscIntNeverNeededParam
  Discrete-Time Integrator1 : DiscreteIntegrator  InitialConditionSource=external  ICPrevOutput=DiscIntNeverNeededParam  ICPrevScaledInput=DiscIntNeverNeededParam
  Mux : Mux  Inputs=2
  Product{1..4} (4 alike) : Product  RndMeth=Zero
  kMtState : Subsystem
  LkMt : Outport
  tag scope: kMt11=global
  wires:
  Fk/1 -> kMtState/2(Fspr)
  kMtState/2(RLeft) -> Product2/1
  Product1/1 -> Add/1
  Product2/1 -> Add/2
  Product3/1 -> Add1/2
  Product4/1 -> Add1/1
  kMtState/4(RRight) -> Product3/1
  kMtState/1(CLeft) -> Product1/1
  Add/1 -> Discrete-Time Integrator/1  "glkMt"
  Add1/1 -> Discrete-Time Integrator1/1  "grkMt"
  Discrete-Time Integrator1/1 -> Add2/2, kMtState/3(LrkMt), Mux/2
  Discrete-Time Integrator/1 -> Add2/1, kMtState/1(LlkMt), Mux/1
  Add2/1 -> LkMt/1
  kMtState/3(CRight) -> Product4/1
  [Rgro] -> Product2/2, Product3/2
  [Rshr] -> Product1/2, Product4/2
  Mux/1 -> [kMt11]
  [LkMt] -> Discrete-Time Integrator/2
  [LkMt] -> Discrete-Time Integrator1/2

== system Coupled_Model_crosslinked_intext/kMtcontrol/kMtcontrol2/kMt Dynamics ==
  Fk : Inport
  Add : Sum  Inputs=-+
  Add1 : Sum  Inputs=-+
  Add2 : Sum
  Discrete-Time Integrator : DiscreteIntegrator  InitialConditionSource=external  ICPrevOutput=DiscIntNeverNeededParam  ICPrevScaledInput=DiscIntNeverNeededParam
  Discrete-Time Integrator1 : DiscreteIntegrator  InitialConditionSource=external  ICPrevOutput=DiscIntNeverNeededParam  ICPrevScaledInput=DiscIntNeverNeededParam
  Mux : Mux  Inputs=2
  Product{1..4} (4 alike) : Product  RndMeth=Zero
  kMtState : Subsystem
  LkMt : Outport
  tag scope: kMt9=global
  wires:
  Fk/1 -> kMtState/2(Fspr)
  kMtState/2(RLeft) -> Product2/1
  Product1/1 -> Add/1
  Product2/1 -> Add/2
  Product3/1 -> Add1/2
  Product4/1 -> Add1/1
  kMtState/4(RRight) -> Product3/1
  kMtState/1(CLeft) -> Product1/1
  Add/1 -> Discrete-Time Integrator/1  "glkMt"
  Add1/1 -> Discrete-Time Integrator1/1  "grkMt"
  Discrete-Time Integrator1/1 -> Add2/2, kMtState/3(LrkMt), Mux/2
  Discrete-Time Integrator/1 -> Add2/1, kMtState/1(LlkMt), Mux/1
  Add2/1 -> LkMt/1
  kMtState/3(CRight) -> Product4/1
  [Rgro] -> Product2/2, Product3/2
  [Rshr] -> Product1/2, Product4/2
  Mux/1 -> [kMt9]
  [LkMt] -> Discrete-Time Integrator/2
  [LkMt] -> Discrete-Time Integrator1/2

== system Coupled_Model_crosslinked_intext/kMtcontrol/kMtcontrol2/kMt Dynamics  ==
  Fk : Inport
  Add : Sum  Inputs=-+
  Add1 : Sum  Inputs=-+
  Add2 : Sum
  Discrete-Time Integrator : DiscreteIntegrator  InitialConditionSource=external  ICPrevOutput=DiscIntNeverNeededParam  ICPrevScaledInput=DiscIntNeverNeededParam
  Discrete-Time Integrator1 : DiscreteIntegrator  InitialConditionSource=external  ICPrevOutput=DiscIntNeverNeededParam  ICPrevScaledInput=DiscIntNeverNeededParam
  Mux : Mux  Inputs=2
  Product{1..4} (4 alike) : Product  RndMeth=Zero
  kMtState : Subsystem
  LkMt : Outport
  tag scope: kMt10=global
  wires:
  Fk/1 -> kMtState/2(Fspr)
  kMtState/2(RLeft) -> Product2/1
  Product1/1 -> Add/1
  Product2/1 -> Add/2
  Product3/1 -> Add1/2
  Product4/1 -> Add1/1
  kMtState/4(RRight) -> Product3/1
  kMtState/1(CLeft) -> Product1/1
  Add/1 -> Discrete-Time Integrator/1  "glkMt"
  Add1/1 -> Discrete-Time Integrator1/1  "grkMt"
  Discrete-Time Integrator1/1 -> Add2/2, kMtState/3(LrkMt), Mux/2
  Discrete-Time Integrator/1 -> Add2/1, kMtState/1(LlkMt), Mux/1
  Add2/1 -> LkMt/1
  kMtState/3(CRight) -> Product4/1
  [Rgro] -> Product2/2, Product3/2
  [Rshr] -> Product1/2, Product4/2
  Mux/1 -> [kMt10]
  [LkMt] -> Discrete-Time Integrator/2
  [LkMt] -> Discrete-Time Integrator1/2

== system Coupled_Model_crosslinked_intext/kMtcontrol/kMtcontrol2/kMt Dynamics   ==
  Fk : Inport
  Add : Sum  Inputs=-+
  Add1 : Sum  Inputs=-+
  Add2 : Sum
  Discrete-Time Integrator : DiscreteIntegrator  InitialConditionSource=external  ICPrevOutput=DiscIntNeverNeededParam  ICPrevScaledInput=DiscIntNeverNeededParam
  Discrete-Time Integrator1 : DiscreteIntegrator  InitialConditionSource=external  ICPrevOutput=DiscIntNeverNeededParam  ICPrevScaledInput=DiscIntNeverNeededParam
  Mux : Mux  Inputs=2
  Product{1..4} (4 alike) : Product  RndMeth=Zero
  kMtState : Subsystem
  LkMt : Outport
  tag scope: kMt12=global
  wires:
  Fk/1 -> kMtState/2(Fspr)
  kMtState/2(RLeft) -> Product2/1
  Product1/1 -> Add/1
  Product2/1 -> Add/2
  Product3/1 -> Add1/2
  Product4/1 -> Add1/1
  kMtState/4(RRight) -> Product3/1
  kMtState/1(CLeft) -> Product1/1
  Add/1 -> Discrete-Time Integrator/1  "glkMt"
  Add1/1 -> Discrete-Time Integrator1/1  "grkMt"
  Discrete-Time Integrator1/1 -> Add2/2, kMtState/3(LrkMt), Mux/2
  Discrete-Time Integrator/1 -> Add2/1, kMtState/1(LlkMt), Mux/1
  Add2/1 -> LkMt/1
  kMtState/3(CRight) -> Product4/1
  [Rgro] -> Product2/2, Product3/2
  [Rshr] -> Product1/2, Product4/2
  Mux/1 -> [kMt12]
  [LkMt] -> Discrete-Time Integrator/2
  [LkMt] -> Discrete-Time Integrator1/2

== system Coupled_Model_crosslinked_intext/kMtcontrol/kMtcontrol3/ Crosslinking   ==
  Spring -1 : Inport
  Spring 0 : Inport  Port=2
  Spring +1 : Inport  Port=3
  F : Inport  Port=4
  xlink K : Inport  Port=5
  Product : Product  RndMeth=Zero
  Product1 : Product  RndMeth=Zero
  Subtract1 : Sum  Inputs=+-
  Subtract3 : Sum  Inputs=-++
  Subtract4 : Sum  Inputs=+-
  Fk crosslink : Outport
  wires:
  Spring -1/1 -> Subtract1/1
  Spring 0/1 -> Subtract1/2, Subtract4/1
  Spring +1/1 -> Subtract4/2
  xlink K/1 -> Product/2, Product1/1
  Subtract1/1 -> Product/1
  Subtract4/1 -> Product1/2
  Product/1 -> Subtract3/1
  F/1 -> Subtract3/2
  Product1/1 -> Subtract3/3
  Subtract3/1 -> Fk crosslink/1

== system Coupled_Model_crosslinked_intext/kMtcontrol/kMtcontrol3/Crosslinking  ==
  Spring -1 : Inport
  Spring 0 : Inport  Port=2
  Spring +1 : Inport  Port=3
  F : Inport  Port=4
  xlink K : Inport  Port=5
  Product : Product  RndMeth=Zero
  Product1 : Product  RndMeth=Zero
  Subtract1 : Sum  Inputs=+-
  Subtract3 : Sum  Inputs=-++
  Subtract4 : Sum  Inputs=+-
  Fk crosslink : Outport
  wires:
  Spring -1/1 -> Subtract1/1
  Spring 0/1 -> Subtract1/2, Subtract4/1
  Spring +1/1 -> Subtract4/2
  xlink K/1 -> Product/2, Product1/1
  Subtract1/1 -> Product/1
  Subtract4/1 -> Product1/2
  Product/1 -> Subtract3/1
  F/1 -> Subtract3/2
  Product1/1 -> Subtract3/3
  Subtract3/1 -> Fk crosslink/1

== system Coupled_Model_crosslinked_intext/kMtcontrol/kMtcontrol3/Crosslinking   ==
  Spring -1 : Inport
  Spring 0 : Inport  Port=2
  Spring +1 : Inport  Port=3
  F : Inport  Port=4
  xlink K : Inport  Port=5
  Product : Product  RndMeth=Zero
  Product1 : Product  RndMeth=Zero
  Subtract1 : Sum  Inputs=+-
  Subtract3 : Sum  Inputs=-++
  Subtract4 : Sum  Inputs=+-
  Fk crosslink : Outport
  wires:
  Spring -1/1 -> Subtract1/1
  Spring 0/1 -> Subtract1/2, Subtract4/1
  Spring +1/1 -> Subtract4/2
  xlink K/1 -> Product/2, Product1/1
  Subtract1/1 -> Product/1
  Subtract4/1 -> Product1/2
  Product/1 -> Subtract3/1
  F/1 -> Subtract3/2
  Product1/1 -> Subtract3/3
  Subtract3/1 -> Fk crosslink/1

== system Coupled_Model_crosslinked_intext/kMtcontrol/kMtcontrol3/Crosslinking    ==
  Spring -1 : Inport
  Spring 0 : Inport  Port=2
  Spring +1 : Inport  Port=3
  F : Inport  Port=4
  xlink K : Inport  Port=5
  Product : Product  RndMeth=Zero
  Product1 : Product  RndMeth=Zero
  Subtract1 : Sum  Inputs=+-
  Subtract3 : Sum  Inputs=-++
  Subtract4 : Sum  Inputs=+-
  Fk crosslink : Outport
  wires:
  Spring -1/1 -> Subtract1/1
  Spring 0/1 -> Subtract1/2, Subtract4/1
  Spring +1/1 -> Subtract4/2
  xlink K/1 -> Product/2, Product1/1
  Subtract1/1 -> Product/1
  Subtract4/1 -> Product1/2
  Product/1 -> Subtract3/1
  F/1 -> Subtract3/2
  Product1/1 -> Subtract3/3
  Subtract3/1 -> Fk crosslink/1

== system Coupled_Model_crosslinked_intext/kMtcontrol/kMtcontrol3/kMt  Dynamics ==
  Fk : Inport
  Add : Sum  Inputs=-+
  Add1 : Sum  Inputs=-+
  Add2 : Sum
  Discrete-Time Integrator : DiscreteIntegrator  InitialConditionSource=external  ICPrevOutput=DiscIntNeverNeededParam  ICPrevScaledInput=DiscIntNeverNeededParam
  Discrete-Time Integrator1 : DiscreteIntegrator  InitialConditionSource=external  ICPrevOutput=DiscIntNeverNeededParam  ICPrevScaledInput=DiscIntNeverNeededParam
  Mux : Mux  Inputs=2
  Product{1..4} (4 alike) : Product  RndMeth=Zero
  kMtState : Subsystem
  LkMt : Outport
  tag scope: kMt15=global
  wires:
  Fk/1 -> kMtState/2(Fspr)
  kMtState/2(RLeft) -> Product2/1
  Product1/1 -> Add/1
  Product2/1 -> Add/2
  Product3/1 -> Add1/2
  Product4/1 -> Add1/1
  kMtState/4(RRight) -> Product3/1
  kMtState/1(CLeft) -> Product1/1
  Add/1 -> Discrete-Time Integrator/1  "glkMt"
  Add1/1 -> Discrete-Time Integrator1/1  "grkMt"
  Discrete-Time Integrator1/1 -> Add2/2, kMtState/3(LrkMt), Mux/2
  Discrete-Time Integrator/1 -> Add2/1, kMtState/1(LlkMt), Mux/1
  Add2/1 -> LkMt/1
  kMtState/3(CRight) -> Product4/1
  [Rgro] -> Product2/2, Product3/2
  [Rshr] -> Product1/2, Product4/2
  Mux/1 -> [kMt15]
  [LkMt] -> Discrete-Time Integrator/2
  [LkMt] -> Discrete-Time Integrator1/2
